simulink model "mInhWithConstTop"  (Simulink 8.0)
settings: Solver=FixedStepDiscrete  StartTime=0.0  StopTime=1  FixedStep=Auto  RelTol=1e-3  SampleTimeConstraint=STIndependent
settings Model: FPTRunName=Active  Creator=The MathWorks Inc.  LastModifiedBy=mtocci  ExtModeAutoUpdateStatusClock=off
settings DataIOCC: SignalLoggingSaveFormat=ModelDataLogs  SignalLoggingName=logsOut
settings OptimizationCC: InlineParams=on  InlineInvariantSignals=on  InitFltsAndDblsToZero=on
settings DebuggingCC: SaveWithParameterizedLinksMsg=none  CheckExecutionContextPreStartOutputMsg=on  CheckExecutionContextRuntimeOutputMsg=on  SolverPrmCheckMsg=none  MultiTaskDSMMsg=warning  MultiTaskCondExecSysMsg=none  SigSpecEnsureSampleTimeMsg=none  FcnCallInpInsideContextMsg=Use local settings  StrictBusMsg=ErrorOnBusTreatedAsVector
settings HardwareCC: TargetHWDeviceType=32-bit Generic
settings ModelReferenceCC: UpdateModelReferenceTargets=IfOutOfDate  CheckModelReferenceTargetMessage=none
settings RTWCC: GenerateReport=on  ProcessScript=grt_make_rtw_hook  LaunchReport=on  IncludeERTFirstTime=on
settings CodeAppCC: MaxIdLength=100
settings GRTTargetCC: TargetFcnLib=ansi_tfl_tmw.mat  SharedFunctionMode=Off  CombineOutputUpdateFcns=off

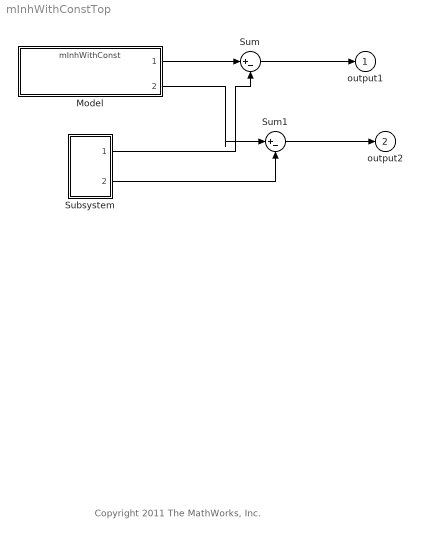
== system mInhWithConstTop ==
  note: Copyright 2011 The MathWorks, Inc.
  Model : ModelReference  ModelNameDialog=mInhWithConst  SimulationMode=Accelerator  ModelReferenceVersion=1.79  CopyOfModelName=mInhWithConst  DefaultDataLogging=on
  Subsystem : Subsystem
  Sum : Sum  Inputs=|+-
  Sum1 : Sum  Inputs=|+-
  output1 : Outport
  output2 : Outport  Port=2
  wires:
  Subsystem/1(output3) -> Sum/2
  Model/1 -> Sum/1
  Sum/1 -> output1/1
  Model/2 -> Sum1/1
  Subsystem/2(output4) -> Sum1/2
  Sum1/1 -> output2/1

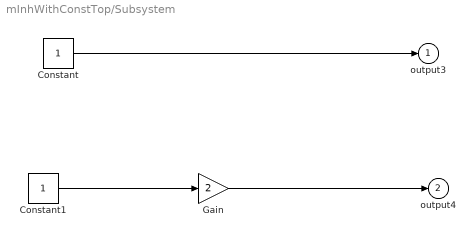
== system mInhWithConstTop/Subsystem ==
  Constant : Constant
  Constant1 : Constant  SampleTime=-1
  Gain : Gain  Gain=2
  output3 : Outport
  output4 : Outport  Port=2
  wires:
  Constant/1 -> output3/1
  Constant1/1 -> Gain/1
  Gain/1 -> output4/1
